simulink library "variableRadiusBasisParams_cl"  (R2018b)
settings: Solver=VariableStepAuto  StartTime=0.0  StopTime=10.0  RelTol=1e-3
undefined symbols (not defined in the file or in its folder): initializeBussesFromBlock
settings Model: Creator=mcobb  LastModifiedBy=mcobb

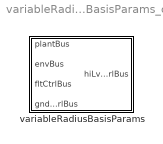
== system variableRadiusBasisParams_cl ==
  variableRadiusBasisParams : Subsystem  LoadFcn=initializeBussesFromBlock(gcb)  InitFcn=initializeBussesFromBlock(gcb)  StartFcn=initializeBussesFromBlock(gcb)  mask{basisParams=[1 1 1]}
      mask prompts: basisParams "Basis Parameters"

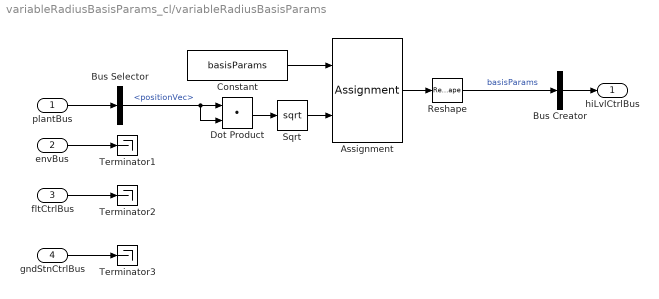
== system variableRadiusBasisParams_cl/variableRadiusBasisParams ==
  plantBus : Inport  OutDataTypeStr=Bus: plantBus
  envBus : Inport  Port=2  OutDataTypeStr=Bus: envBus
  fltCtrlBus : Inport  Port=3  OutDataTypeStr=Bus: fltCtrlBus
  gndStnCtrlBus : Inport  Port=4  OutDataTypeStr=Bus: gndStnCtrlBus
  Assignment : Assignment  DiagnosticForDimensions=Warning  IndexOptions=Index vector (dialog)  Indices=numel(basisParams)  OutputSizes=1
  Bus Creator : BusCreator  Inputs=1  OutDataTypeStr=Bus: hiLvlCtrlBus
  Bus Selector : BusSelector  OutputSignals=positionVec
  Constant : Constant  Value=basisParams
  Dot Product : DotProduct  InputSameDT=on  OutDataTypeStr=Inherit: Inherit via internal rule
  Reshape : Reshape  OutputDimensionality=Column vector (2-D)
  Sqrt : Sqrt  SaturateOnIntegerOverflow=on
  Terminator1 : Terminator
  Terminator2 : Terminator
  Terminator3 : Terminator
  hiLvlCtrlBus : Outport  OutDataTypeStr=Bus: hiLvlCtrlBus
  wires:
  envBus/1 -> Terminator1/1
  gndStnCtrlBus/1 -> Terminator3/1
  Bus Creator/1 -> hiLvlCtrlBus/1
  Constant/1 -> Assignment/1
  fltCtrlBus/1 -> Terminator2/1
  plantBus/1 -> Bus Selector/1
  Reshape/1 -> Bus Creator/1  "basisParams"
  Bus Selector/1 -> Dot Product/2, Dot Product/1  "<positionVec>"
  Dot Product/1 -> Sqrt/1
  Sqrt/1 -> Assignment/2
  Assignment/1 -> Reshape/1
